simulink model "Braking_ABS_V3"  (R2023b)
settings: Solver=VariableStepAuto  StartTime=0.0  StopTime=3  RelTol=1e-3
values from neighbouring files (symbols this model uses):
  A = 2    [Braking_Param.m]
  c1 = 0.86    [Braking_Param.m]
  c2 = 33.82    [Braking_Param.m]
  c3 = 0.36    [Braking_Param.m]
  cw = 0.3    [Braking_Param.m]
  g = 9.81    [Braking_Param.m]
  Jw = 0.8    [Braking_Param.m]
  Kc = 20000    [Braking_Param.m]
  m = 1500    [Braking_Param.m]
  p = 1.2    [Braking_Param.m]
  rw = 0.3    [Braking_Param.m]
  v0 = 100/3.6    (= 27.7777777778)    [Braking_Param.m]
libraries: simulink x2
settings Model: Creator=34266  LastModifiedBy=BeanieBabyJ
settings SolverCC: ZeroCrossAlgorithm=Adaptive
settings DebuggingCC: IgnoredZcDiagnostic=none

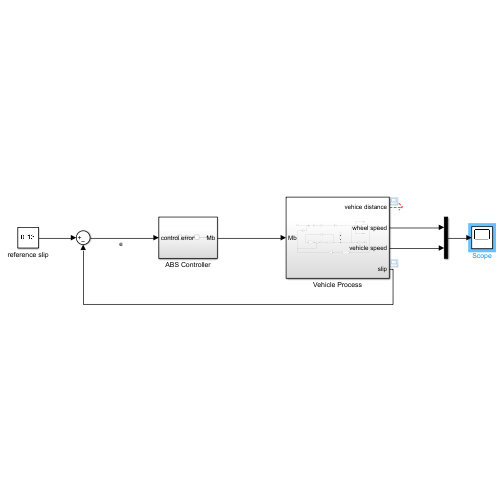
[thumbnail: Simulink's stored preview of the top-level diagram]
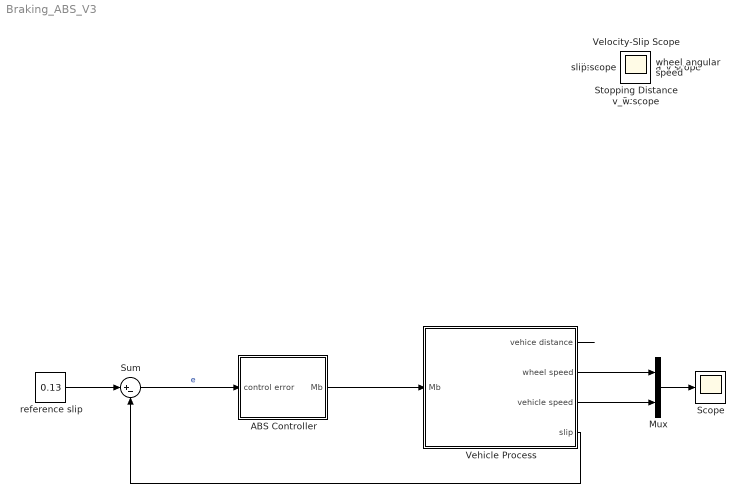
== system Braking_ABS_V3 ==
  ABS Controller : Subsystem
  Mux : Mux  Inputs=2
  Scope : Scope
  Sum : Sum  Inputs=|+-
  Vehicle Process : Subsystem
  reference slip : Constant  Value=0.13
  Stopping Distance Scope : Scope
  Velocity-Slip Scope : Scope
  a_v scope : Scope
  distance : Scope
  slip scope : Scope
  v_w scope : Scope
  wheel angular speed : Scope
  wires:
  ABS Controller/1(Mb) -> Vehicle Process/1(Mb)
  Vehicle Process/1(vehice distance) -> ?
  reference slip/1 -> Sum/1
  Vehicle Process/4(slip) -> Sum/2
  Sum/1 -> ABS Controller/1(control error)  "e"
  Vehicle Process/2(wheel speed) -> Mux/1
  Vehicle Process/3(vehicle speed) -> Mux/2
  Mux/1 -> Scope/1

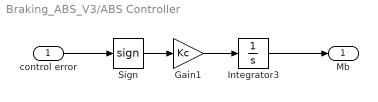
== system Braking_ABS_V3/ABS Controller ==
  control error : Inport
  Gain1 : Gain  Gain=Kc
  Integrator3 : Integrator  LimitOutput=on  LowerSaturationLimit=0  ZeroCross=off
  Sign : Signum
  Mb : Outport
  wires:
  Integrator3/1 -> Mb/1
  control error/1 -> Sign/1
  Gain1/1 -> Integrator3/1
  Sign/1 -> Gain1/1

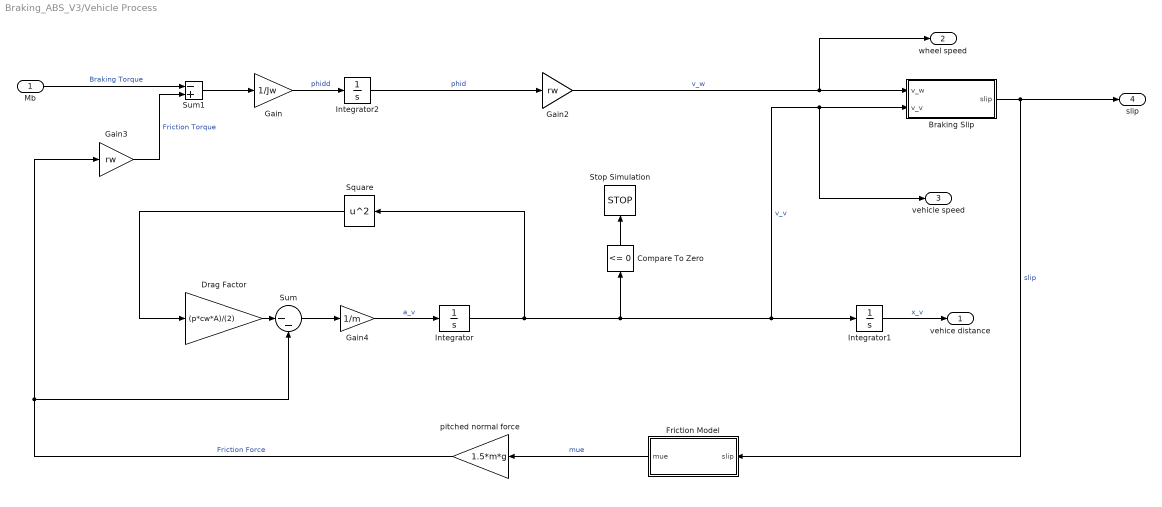
== system Braking_ABS_V3/Vehicle Process ==
  Mb : Inport
  Braking Slip : Subsystem
  Compare To Zero : simulink/Logic and Bit Operations/Compare To Zero  relop=<=  OutDataTypeStr=boolean
  Drag Factor : Gain  Gain=(p*cw*A)/(2)
  Friction Model : Subsystem
  Gain : Gain  Gain=1/Jw
  Gain2 : Gain  Gain=rw
  Gain3 : Gain  Gain=rw
  Gain4 : Gain  Gain=1/m
  Integrator : Integrator  InitialCondition=v0  LimitOutput=on  LowerSaturationLimit=0
  Integrator1 : Integrator  LimitOutput=on  LowerSaturationLimit=0
  Integrator2 : Integrator  InitialCondition=v0/rw  LimitOutput=on  LowerSaturationLimit=0
  Square : Math  Operator=square
  Stop Simulation : Stop
  Sum : Sum  Inputs=|--
  Sum1 : Sum  Inputs=-+
  pitched normal force : Gain  Gain=1.5*m*g
  vehice distance : Outport
  wheel speed : Outport  Port=2
  vehicle speed : Outport  Port=3
  slip : Outport  Port=4
  wires:
  Braking Slip/1(slip) -> Friction Model/1(slip), slip/1  "slip"
  Integrator/1 -> Square/1, vehicle speed/1, Braking Slip/2(v_v), Integrator1/1, Compare To Zero/1  "v_v"
  Friction Model/1(mue) -> pitched normal force/1  "mue"
  Compare To Zero/1 -> Stop Simulation/1
  pitched normal force/1 -> Sum/2, Gain3/1  "Friction Force"
  Gain/1 -> Integrator2/1  "phidd"
  Integrator2/1 -> Gain2/1  "phid"
  Sum/1 -> Gain4/1
  Drag Factor/1 -> Sum/1
  Square/1 -> Drag Factor/1
  Gain2/1 -> wheel speed/1, Braking Slip/1(v_w)  "v_w"
  Gain3/1 -> Sum1/2  "Friction Torque"
  Sum1/1 -> Gain/1
  Gain4/1 -> Integrator/1  "a_v"
  Integrator1/1 -> vehice distance/1  "x_v"
  Mb/1 -> Sum1/1  "Braking Torque"

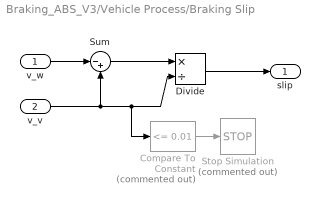
== system Braking_ABS_V3/Vehicle Process/Braking Slip ==
  v_w : Inport
  v_v : Inport  Port=2
  Compare To Constant : simulink/Logic and Bit Operations/Compare To Constant  Commented=on  relop=<=  const=0.01  OutDataTypeStr=boolean
  Divide : Product  Inputs=*/
  Stop Simulation : Stop  Commented=on
  Sum : Sum  Inputs=|-+
  slip : Outport
  wires:
  Sum/1 -> Divide/1
  v_v/1 -> Sum/2, Compare To Constant/1, Divide/2
  v_w/1 -> Sum/1
  Divide/1 -> slip/1
  Compare To Constant/1 -> Stop Simulation/1

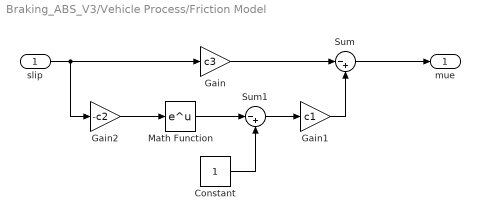
== system Braking_ABS_V3/Vehicle Process/Friction Model ==
  slip : Inport
  Constant : Constant
  Gain : Gain  Gain=c3
  Gain1 : Gain  Gain=c1
  Gain2 : Gain  Gain=-c2
  Math Function : Math
  Sum : Sum  Inputs=|-+
  Sum1 : Sum  Inputs=|-+
  mue : Outport
  wires:
  Sum1/1 -> Gain1/1
  slip/1 -> Gain/1, Gain2/1
  Gain2/1 -> Math Function/1
  Math Function/1 -> Sum1/1
  Constant/1 -> Sum1/2
  Gain1/1 -> Sum/2
  Gain/1 -> Sum/1
  Sum/1 -> mue/1
